simulink model "RCcircuit"  (R2017a)
settings: Solver=VariableStepAuto  StartTime=0.0  StopTime=2  RelTol=1e-3
values from neighbouring files (symbols this model uses):
  C = 10e-6    (= 1e-05)    [RCcircuit.m]
  Freq = 1    [RCcircuit.m]
  R = 10e3    (= 10000)    [RCcircuit.m]
libraries: simulink x1
settings Model: Creator=jms2299  LastModifiedBy=jms2299

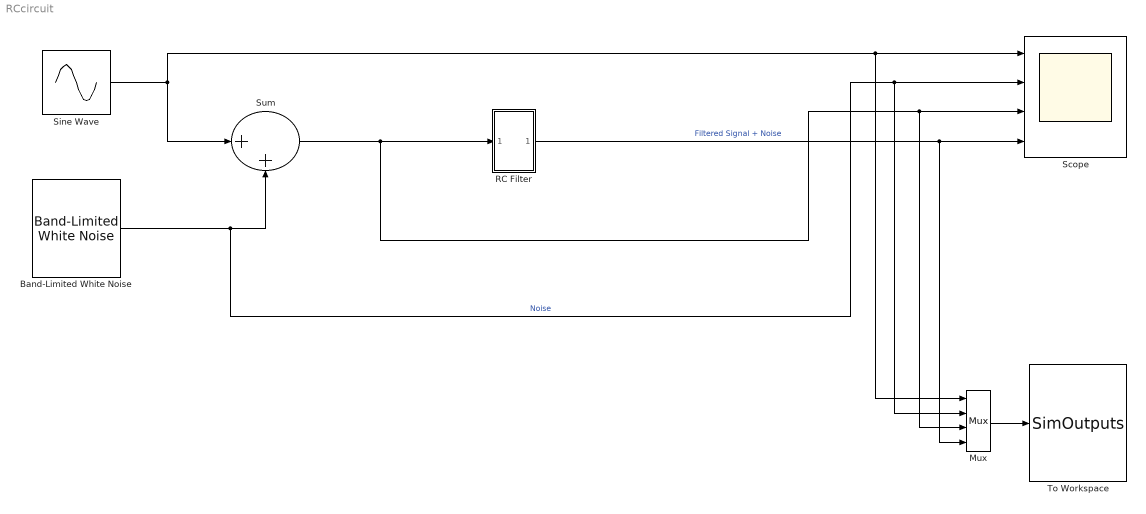
== system RCcircuit ==
  Band-Limited White Noise : simulink/Sources/Band-Limited White Noise  Cov=[0.001]  Ts=0.001  seed=[23341]
  Mux : Mux
  RC Filter : Subsystem
  Scope : Scope  NumInputPorts=4
  Sine Wave : Sin  Frequency=2*pi*Freq  SampleTime=0
  Sum : Sum  Inputs=|++
  To Workspace : ToWorkspace  VariableName=SimOutputs  SampleTime=-1
  wires:
  Sine Wave/1 -> Sum/1, Mux/1, Scope/1
  RC Filter/1(Vout) -> Mux/4, Scope/4  "Filtered Signal + Noise"
  Band-Limited White Noise/1 -> Mux/2, Scope/2, Sum/2  "Noise"
  Sum/1 -> Mux/3, Scope/3, RC Filter/1(Vin)
  Mux/1 -> To Workspace/1

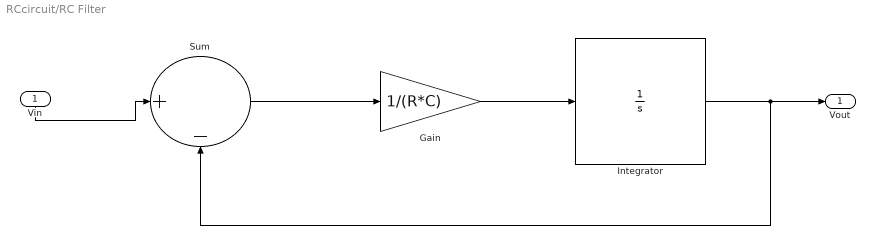
== system RCcircuit/RC Filter ==
  Vin : Inport
  Gain : Gain  Gain=1/(R*C)
  Integrator : Integrator
  Sum : Sum  Inputs=|+-
  Vout : Outport
  wires:
  Gain/1 -> Integrator/1
  Sum/1 -> Gain/1
  Vin/1 -> Sum/1
  Integrator/1 -> Sum/2, Vout/1
